simulink model "tyreModelTest"  (R2013b)
settings: Solver=ode45  StartTime=0.0  StopTime=200.0  RelTol=1e-3
libraries: simulink x1
settings Model: Creator=lasse  LastModifiedBy=lasse

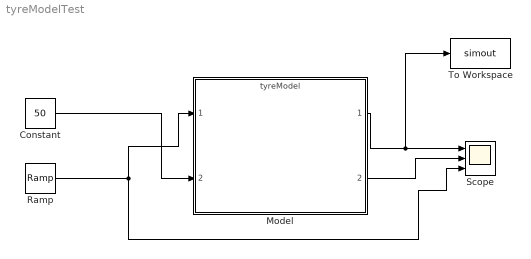
== system tyreModelTest ==
  Constant : Constant  Value=50
  Model : ModelReference  ModelNameDialog=tyreModel.slx  SimulationMode=Normal  ModelReferenceVersion=1.26  CopyOfModelName=tyreModel.slx  DefaultDataLogging=on
  Ramp : simulink/Sources/Ramp  slope=1  start=0  X0=-100
  Scope : Scope  NumInputPorts=3
      settings: YMin=-5~-5~-5  YMax=5~5~5
  To Workspace : ToWorkspace  VariableName=simout  SampleTime=-1  SaveFormat=Timeseries
  wires:
  Model/1 -> To Workspace/1, Scope/1
  Model/2 -> Scope/2
  Ramp/1 -> Scope/3, Model/1
  Constant/1 -> Model/2
